simulink model "untitled"  (R2013a)
settings: Solver=ode45  StartTime=0.0  StopTime=100.0  RelTol=1e-3
undefined symbols (not defined in the file or in its folder): sigbuilder_block
settings Model: Creator=USER  LastModifiedBy=USER

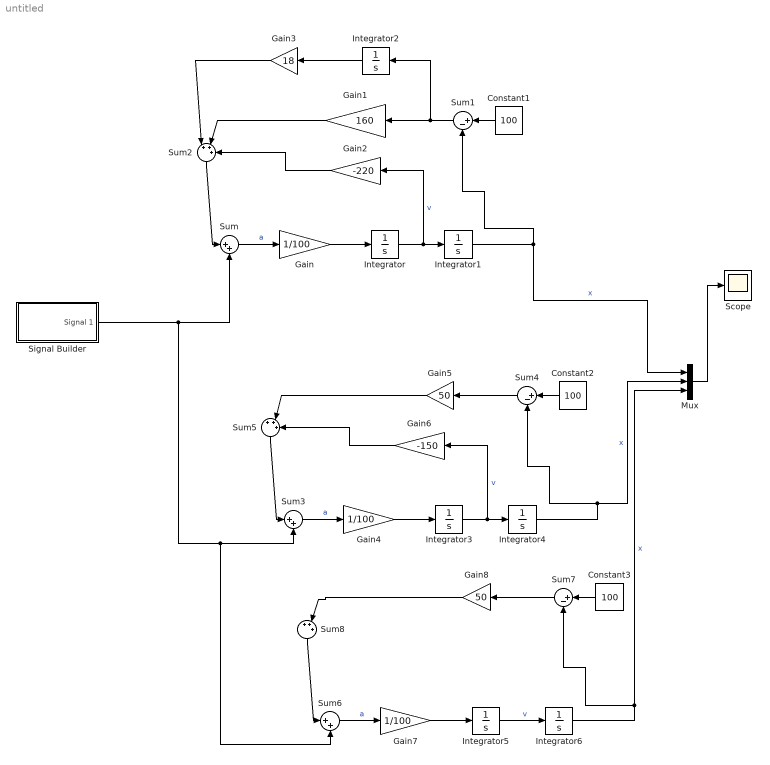
== system untitled ==
  Constant1 : Constant  Value=100
  Constant2 : Constant  Value=100
  Constant3 : Constant  Value=100
  Gain : Gain  Gain=1/100
  Gain1 : Gain  Gain=160
  Gain2 : Gain  Gain=-220
  Gain3 : Gain  Gain=18
  Gain4 : Gain  Gain=1/100
  Gain5 : Gain  Gain=50
  Gain6 : Gain  Gain=-150
  Gain7 : Gain  Gain=1/100
  Gain8 : Gain  Gain=50
  Integrator : Integrator  InitialCondition=20
  Integrator{1..2,4,6} (4 alike) : Integrator  InitialCondition=-80
  Integrator3 : Integrator  InitialCondition=20
  Integrator5 : Integrator  InitialCondition=20
  Mux : Mux  Inputs=3
  Scope : Scope
  Signal Builder : Subsystem  Tag=STV Subsys  LoadFcn=sigbuilder_block('load');  StartFcn=sigbuilder_block('start');  StopFcn=sigbuilder_block('stop');  ClipboardFcn=sigbuilder_block('clipboard');  mask(Sigbuilder block){}
      mask help: Simulink:masks:SigbuilderBlock_MD
      mask init:
      | if ~strcmp(get_param(bdroot(gcbh),'SimulationStatus'),'stopped') tuvar = sigbuilder_block('maskInit'); end
      settings: CopyFcn=sigbuilder_block('copy');  DeleteFcn=sigbuilder_block('delete');  ModelCloseFcn=sigbuilder_block('modelClose');  PreSaveFcn=sigbuilder_block('preSave');  PauseFcn=sigbuilder_block('pause');  ContinueFcn=sigbuilder_block('continue');  NameChangeFcn=sigbuilder_block('namechange');  OpenFcn=sigbuilder_block('open',[321.75 64.5 550.5 394.5 ]);  CloseFcn=sigbuilder_block('close');
      mask Display: plot(0, 0, 100, 100,[2, 2, 32, 32, 2], [68, 8, 8, 68, 68],[32, 2], [38, 38], [32, 19, 2],[53, 60, 44], [32, 17, 17, 2],[16, 16, 31, 31]);txt = getActiveGroup(gcbh);text(2, 100, txt,'verticalAlignment', 'top');
  Sum : Sum  Inputs=|++
  Sum1 : Sum  Inputs=|+-
  Sum2 : Sum  Inputs=|+++
  Sum3 : Sum  Inputs=|++
  Sum4 : Sum  Inputs=|+-
  Sum5 : Sum  Inputs=|+++
  Sum6 : Sum  Inputs=|++
  Sum7 : Sum  Inputs=|+-
  Sum8 : Sum  Inputs=|+++
  wires:
  Gain/1 -> Integrator/1
  Sum/1 -> Gain/1  "a"
  Integrator/1 -> Gain2/1, Integrator1/1  "v"
  Sum1/1 -> Integrator2/1, Gain1/1
  Constant1/1 -> Sum1/1
  Integrator1/1 -> Sum1/2, Mux/1  "x"
  Sum2/1 -> Sum/1
  Gain1/1 -> Sum2/2
  Gain2/1 -> Sum2/3
  Integrator2/1 -> Gain3/1
  Gain3/1 -> Sum2/1
  Gain4/1 -> Integrator3/1
  Sum3/1 -> Gain4/1  "a"
  Integrator3/1 -> Gain6/1, Integrator4/1  "v"
  Sum4/1 -> Gain5/1
  Constant2/1 -> Sum4/1
  Integrator4/1 -> Mux/2, Sum4/2  "x"
  Sum5/1 -> Sum3/1
  Gain5/1 -> Sum5/2
  Gain6/1 -> Sum5/3
  Signal Builder/1(Signal 1) -> Sum3/2, Sum6/2, Sum/2
  Gain7/1 -> Integrator5/1
  Sum6/1 -> Gain7/1  "a"
  Integrator5/1 -> Integrator6/1  "v"
  Sum7/1 -> Gain8/1
  Constant3/1 -> Sum7/1
  Integrator6/1 -> Mux/3, Sum7/2  "x"
  Sum8/1 -> Sum6/1
  Gain8/1 -> Sum8/2
  Mux/1 -> Scope/1

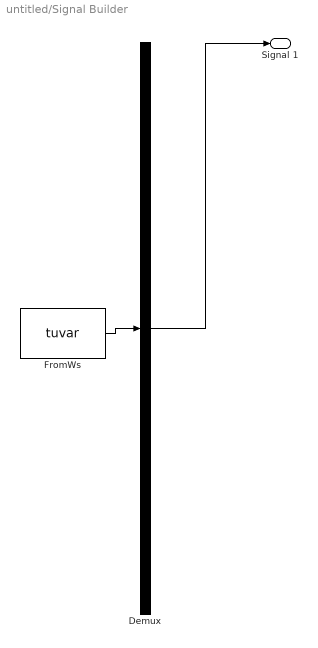
== system untitled/Signal Builder ==
  Demux : Demux  Tag=STV Demux  Outputs=1
  FromWs : FromWorkspace  Tag=STV FromWs  VariableName=tuvar  SampleTime=0
      SigBuilderData=|
      | common.afterFinalStr = 'Extrapolate'
      | common.sampleTime = 0
      | dataSet.timeRange = [0 100]
      | dataSet.name = 'Group 1'
      | sbobj.Groups.Name = 'Group 1'
      | sbobj.Groups.Signals.Name = 'Signal 1'
      | sbobj.Groups.Signals.XData = [0 60.2 60.2 79.8 79.8 100]
      | sbobj.Groups.Signals.YData = [-1e-06 1e-06 990 990 -1480 -1480]
      | sbobj.Groups.TimeRange = [0 100]
  Signal 1 : Outport  Tag=STV Outport
  wires:
  Demux/1 -> Signal 1/1
  FromWs/1 -> Demux/1
